simulink model "FOC_PMSM"  (Simulink 10.0)
settings: Solver=ode45  StartTime=0  StopTime=10  FixedStep=1/fs/4  MaxStep=1/fs/2  RelTol=1e-7  EnableMultiTasking=on
InitFcn:
  | Motor_parameters_Lsrpm7fw
values from neighbouring files (symbols this model uses):
  c2 = -L2/(L1^2-L2^2)    (= 10.9375)    [Motor_parameters_Lsrpm7fw.m]
  fs = 10e3    (= 10000)    [Motor_parameters_Lsrpm7fw.m]
  Iphmax = I_rated*sqrt(2)*3    [Motor_parameters_Lsrpm7fw.m]
  J = 1*1e-3    (= 0.001)    [Motor_parameters_Lsrpm7fw.m]
  Ki1 = 2    [Motor_parameters_Lsrpm7fw.m]
  Ki2 = 10000    [Motor_parameters_Lsrpm7fw.m]
  Ki_pll = 100    [Motor_parameters_Lsrpm7fw.m]
  Kp1 = 0.05    [Motor_parameters_Lsrpm7fw.m]
  Kp2 = 12    [Motor_parameters_Lsrpm7fw.m]
  Kp_pll = 10    [Motor_parameters_Lsrpm7fw.m]
  Ld = 10e-3    (= 0.01)    [Motor_parameters_Lsrpm7fw.m]
  Lndd_ini = Lndmpm    (= 0.412)    [Motor_parameters_Lsrpm7fw.m]
  Lndmpm = 0.412    [Motor_parameters_Lsrpm7fw.m]
  Lq = 12.8e-3    (= 0.0128)    [Motor_parameters_Lsrpm7fw.m]
  Npp = 8/2    (= 4)    [Motor_parameters_Lsrpm7fw.m]
  Omegae_ini = 0    [Motor_parameters_Lsrpm7fw.m]
  Rs = 0.78    [Motor_parameters_Lsrpm7fw.m]
  Tl_const = Trat/nrat^2    (= 1.24081632653e-05)    [Motor_parameters_Lsrpm7fw.m]
  Trat = 38    [Motor_parameters_Lsrpm7fw.m]
  Vm = 45    [Motor_parameters_Lsrpm7fw.m]
  Vph = Vs*sqrt(2)    [Motor_parameters_Lsrpm7fw.m]
  wo = 10    [Motor_parameters_Lsrpm7fw.m]
undefined symbols (not defined in the file or in its folder): DiscIntNeverNeededParam, sigbuilder_block
libraries: simulink x1
(part 1 of 2)
settings Model: Creator=klu  LastModifiedBy=Kristina
settings DataIOCC: LimitDataPoints=on  SignalLoggingSaveFormat=ModelDataLogs
settings OptimizationCC: BooleanDataType=off  ExpressionDepthLimit=2147483647  InitFltsAndDblsToZero=on
settings DebuggingCC: AlgebraicLoopMsg=none  SaveWithParameterizedLinksMsg=none  SignalResolutionControl=TryResolveAllWithWarning  MultiTaskDSMMsg=warning  MultiTaskCondExecSysMsg=none  FcnCallInpInsideContextMsg=warning  StateNameClashWarn=warning
settings GRTTargetCC: TargetFcnLib=ansi_tfl_tmw.mat  GeneratePreprocessorConditionals=Disable all
settings ConfigComp: CovExternalEMLEnable=off  CovSFcnEnable=off

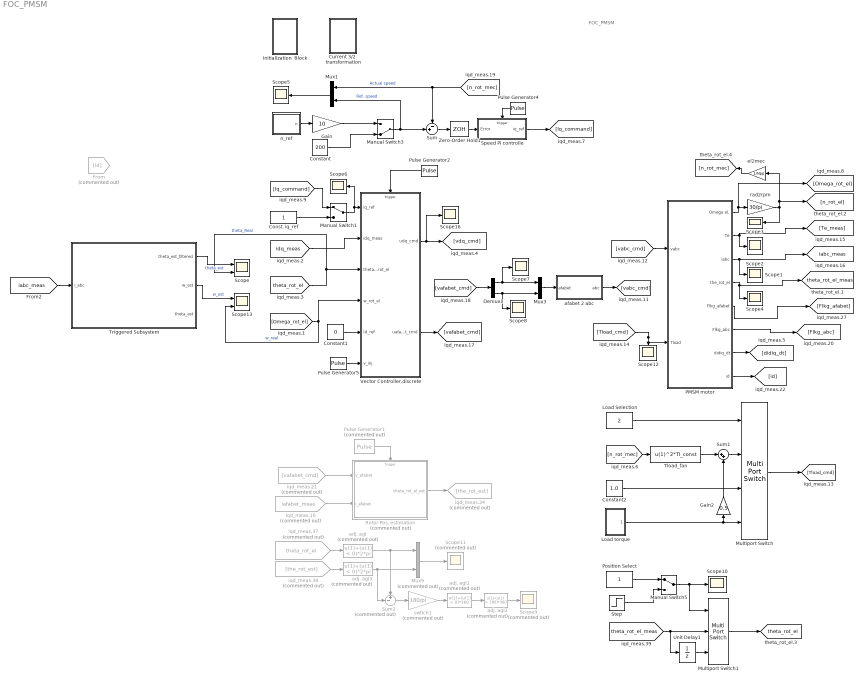
== system FOC_PMSM ==
  note: FOC_PMSM
  Const. iq_ref : Constant
  Constant : Constant  Value=200
  Constant1 : Constant  Value=0
  Constant2 : Constant  Value=1.0
  Current 3/2  transformation : Subsystem
      mask Display:
      | plot([0.1000    0.1357    0.1714    0.2071    0.2429    0.2786    0.3143    0.3500    0.3857    0.4214 0.4571    0.4929    0.5286    0.5643    0.6000]-0.05,0.4+0.6*[0.5000    0.5868    0.6564    0.6950    0.6950    0.6564    0.5868    0.5000    0.4132    0.3436 0.3050    0.3050    0.3436    0.4132    0.5000])
      | 
      | plot([0.1,0.9],[0.1,0.9])
      | 
      | plot([0.5,0.9],0.3*[1 1])
  Demux1 : Demux  Outputs=2
  From : From  Commented=on  GotoTag=id
  Gain : Gain  Gain=10
  Gain2 : Gain  Gain=0.5
  Initialization  Block : Subsystem  mask{init_in=Motor_parameters_Lsrpm7fw}
      mask prompts: init_in "Enter Initialization Script:"
      mask init:
      | aaa =3;
      mask Callback init_in:
      | init_script=get_param(gcb,'MaskValueString');
      | %eval(init_script);
      | %set_param(gcs,'PreLoadFcn',init_script)
      | set_param(gcs,'InitFcn',init_script)
      | 
      | % Change the parameters here;
      | Ld               = Ld;
      | Lq               = Ld;
  Load Selection : Constant  Value=2
  Load torque : Subsystem
  Manual Switch1 : ManualSwitch
  Manual Switch3 : ManualSwitch  CurrentSetting=0
  Manual Switch5 : ManualSwitch
  Multiport Switch : MultiPortSwitch
  Multiport Switch1 : MultiPortSwitch  Inputs=2
  Mux1 : Mux  Inputs=2
  Mux3 : Mux  Inputs=2
  Mux9 : Mux  Commented=on  Inputs=2
  PMSM motor : Subsystem
  Position Select : Constant
  Pulse Generator1 : DiscretePulseGenerator  Commented=on  PulseType=Time based  Period=1/fs  PulseWidth=50  PhaseDelay=1/fs/4*0
  Pulse Generator2 : DiscretePulseGenerator  PulseType=Time based  Period=1/fs  PulseWidth=50
  Pulse Generator4 : DiscretePulseGenerator  PulseType=Time based  Period=1/fs*2  PulseWidth=50
  Pulse Generator5 : DiscretePulseGenerator  PulseType=Time based  Amplitude=Vm  Period=2/fs  PulseWidth=50  PhaseDelay=1/fs
  Rotor Pos. estimation : Subsystem  Commented=on
  Scope : Scope  NumInputPorts=2
  Scope{1..8,10,12,16} (11 alike) : Scope
  Scope11 : Scope  Commented=on
  Scope13 : Scope  NumInputPorts=2
  Scope9 : Scope  Commented=on
  Speed PI controlle : Subsystem
  Step : Step  Time=0  Before=1  After=2  SampleTime=0
  Sum : Sum  Inputs=-+|
  Sum1 : Sum  Inputs=|++
  Sum2 : Sum  Commented=on  Inputs=+-|
  Tload_fan : Fcn  Expr=u(1)^2*Tl_const
  Triggered Subsystem : Subsystem  TreatAsAtomicUnit=on
  Unit Delay1 : UnitDelay  SampleTime=(1/fs)*4  HasFrameUpgradeWarning=on
  Vector Controller.discrete : Subsystem
  Zero-Order Hold1 : ZeroOrderHold  SampleTime=1/5e3
  adj. agl : Fcn  Commented=on  Expr=u(1)+(u(1) < 0)*2*pi
  adj. agl1 : Fcn  Commented=on  Expr=u(1)+(u(1) < 0)*360
  adj. agl2 : Fcn  Commented=on  Expr=u(1)-(u(1) > 180)*360
  adj. agl3 : Fcn  Commented=on  Expr=u(1)+(u(1) < 0)*2*pi
  afabet 2 abc : Subsystem
  el2mec : Gain  Gain=1/Npp
  iqd_meas.10 : From  Commented=on  GotoTag=iafabet_meas  TagVisibility=global
      settings: CloseFcn=tagdialog Close
  iqd_meas.21 : From  Commented=on  GotoTag=vafabet_cmd
      settings: CloseFcn=tagdialog Close
  iqd_meas.34 : Goto  Commented=on  GotoTag=the_rot_est
  iqd_meas.37 : From  Commented=on  GotoTag=theta_rot_el  TagVisibility=global
      settings: CloseFcn=tagdialog Close
  iqd_meas.38 : From  Commented=on  GotoTag=the_rot_est
      settings: CloseFcn=tagdialog Close
  n_ref : Subsystem  Tag=STV Subsys  LoadFcn=sigbuilder_block('load');  StartFcn=sigbuilder_block('start');  StopFcn=sigbuilder_block('stop');  ClipboardFcn=sigbuilder_block('clipboard');  mask(Sigbuilder block){tuvar=[0:10]}
      mask help: Sigbuilder GUI
      mask init:
      | if ~strcmp(get_param(bdroot(gcbh),'SimulationStatus'),'stopped') tuvar = sigbuilder_block('maskInit'); end
      settings: CopyFcn=sigbuilder_block('copy');  DeleteFcn=sigbuilder_block('delete');  ModelCloseFcn=sigbuilder_block('modelClose');  PreSaveFcn=sigbuilder_block('preSave');  PauseFcn=sigbuilder_block('pause')  ContinueFcn=sigbuilder_block('continue')  NameChangeFcn=sigbuilder_block('namechange');  OpenFcn=sigbuilder_block('open',[72.75 116.25 550.5 363.75 ]);  CloseFcn=sigbuilder_block('close');
      mask Display: plot(0, 0, 100, 100,[2, 2, 32, 32, 2], [68, 8, 8, 68, 68],[32, 2], [38, 38], [32, 19, 2],[53, 60, 44], [32, 17, 17, 2],[16, 16, 31, 31]);txt = getActiveGroup(gcbh);text(2, 100, txt,'verticalAlignment', 'top');
  rad2rpm : Gain  Gain=30/pi
  swtich1 : Gain  Commented=on  Gain=180/pi
  tag scope: iabc_meas=global, theta_rot_el=global, theta_rot_el_meas=global
  wires:
  Mux1/1 -> Scope5/1
  Sum/1 -> Zero-Order Hold1/1
  Manual Switch1/1 -> Scope6/1, Vector Controller.discrete/1(iq_ref)
  Const. iq_ref/1 -> Manual Switch1/2
  Zero-Order Hold1/1 -> Speed PI controlle/1(Error)
  Constant/1 -> Manual Switch3/2
  Manual Switch3/1 -> Mux1/2, Sum/2  "Ref. speed"
  [idq_meas] -> Vector Controller.discrete/2(idq_meas)
  Vector Controller.discrete/2(uafabet_cmd) -> [vafabet_cmd]
  [n_rot_mec] -> Mux1/1, Sum/1  "Actual speed"
  Constant2/1 -> Multiport Switch/3
  Load torque/1(T_load) -> Multiport Switch/4, Gain2/1
  Multiport Switch/1 -> [Tload_cmd]
  [n_rot_mec] -> Tload_fan/1
  Load Selection/1 -> Multiport Switch/1
  [theta_rot_el_meas] -> Unit Delay1/1, Multiport Switch1/2
  Multiport Switch1/1 -> [theta_rot_el]
  Position Select/1 -> Manual Switch5/1
  Step/1 -> Manual Switch5/2
  Manual Switch5/1 -> Multiport Switch1/1, Scope10/1
  n_ref/1(n) -> Gain/1
  Gain/1 -> Manual Switch3/1
  Pulse Generator2/1 -> Vector Controller.discrete/Trigger
  Sum1/1 -> Multiport Switch/2
  Tload_fan/1 -> Sum1/1
  Pulse Generator4/1 -> Speed PI controlle/Trigger
  [theta_rot_el] -> Scope/2, Vector Controller.discrete/3(theta_rot_el)  "theta_Real"
  Constant1/1 -> Vector Controller.discrete/5(Id_ref)
  Gain2/1 -> Sum1/2
  Unit Delay1/1 -> Multiport Switch1/3
  [Omega_rot_el] -> Scope13/2, Vector Controller.discrete/4(w_rot_el)  "w_real"
  PMSM motor/2(Te) -> Scope2/1, [Te_meas]
  PMSM motor/1(Omega el.) -> [Omega_rot_el], rad2rpm/1
  [vabc_cmd] -> PMSM motor/1(vabc)
  rad2rpm/1 -> el2mec/1, [n_rot_el], Scope3/1
  PMSM motor/4(the_rot_el) -> Scope4/1, [theta_rot_el_meas]
  PMSM motor/5(Flkg_afabet) -> [Flkg_afabet]
  PMSM motor/6(Flkg_abc) -> [Flkg_abc]
  [Tload_cmd] -> Scope12/1, PMSM motor/2(Tload)
  PMSM motor/3(iabc) -> Scope1/1, [iabc_meas]
  PMSM motor/7(didiq_dt) -> [didiq_dt]
  Demux1/2 -> Mux3/2, Scope8/1
  Demux1/1 -> Scope7/1, Mux3/1
  [vafabet_cmd] -> Demux1/1
  afabet 2 abc/1(abc) -> [vabc_cmd]
  Mux3/1 -> afabet 2 abc/1(afabet)
  el2mec/1 -> [n_rot_mec]
  Speed PI controlle/1(iq_ref) -> [Iq_command]
  [Iq_command] -> Manual Switch1/1
  adj. agl1/1 -> adj. agl2/1
  iqd_meas.38/1 -> adj. agl3/1
  adj. agl2/1 -> Scope9/1
  iqd_meas.10/1 -> Rotor Pos. estimation/2(i_afabet)
  swtich1/1 -> adj. agl1/1
  Sum2/1 -> swtich1/1
  iqd_meas.21/1 -> Rotor Pos. estimation/1(v_afabet)
  Mux9/1 -> Scope11/1
  Rotor Pos. estimation/1(theta_rot_el_est) -> iqd_meas.34/1
  adj. agl/1 -> Mux9/1, Sum2/1
  iqd_meas.37/1 -> adj. agl/1
  Pulse Generator1/1 -> Rotor Pos. estimation/Trigger
  adj. agl3/1 -> Mux9/2, Sum2/2
  PMSM motor/8("id   ") -> [id]
  Triggered Subsystem/2(w_est) -> Scope13/1  "w_est"
  Vector Controller.discrete/1(udq_cmd) -> Scope16/1, [vdq_cmd]
  Triggered Subsystem/1(theta_est_filtered) -> Scope/1  "theta_est"
  Pulse Generator5/1 -> Vector Controller.discrete/6("v_inj ")
  [iabc_meas] -> Triggered Subsystem/1(i_abc)

== system FOC_PMSM/Current 3/2  transformation ==
  Detect peak : Subsystem
  Display : Display
  Display1 : Display
  Manual Switch7 : ManualSwitch  CurrentSetting=0
  Scope14 : Scope
  Scope6 : Scope
  abc 2 dq : Subsystem
  dq 2 afa beta : Subsystem
  tag scope: iafabet_meas=global, idq_meas=global
  wires:
  abc 2 dq/1(dq) -> [idq_meas], Scope6/1, dq 2 afa beta/1(dq)
  dq 2 afa beta/1(afa beta) -> [iafabet_meas], Scope14/1
  Manual Switch7/1 -> abc 2 dq/1(abc), Detect peak/1(iabc)
  Detect peak/1(Peak) -> Display/1
  [theta_rot_el] -> abc 2 dq/2(theta), dq 2 afa beta/2(theta), Display1/1
  [iabc_meas] -> Manual Switch7/1, Manual Switch7/2

== system FOC_PMSM/Initialization  Block ==

== system FOC_PMSM/Load torque ==
  Add : Sum  Inputs=+++
  Scope2 : Scope
  Step Load torque 1 : Step  Time=2  After=Trat  SampleTime=0
  Step Load torque2 : Step  Time=4  After=-Trat/2  SampleTime=0
  Tload : Constant  Value=0
  T_load : Outport  VectorParamsAs1DForOutWhenUnconnected=off
  wires:
  Tload/1 -> Add/1
  Step Load torque 1/1 -> Add/2
  Step Load torque2/1 -> Add/3
  Add/1 -> T_load/1, Scope2/1

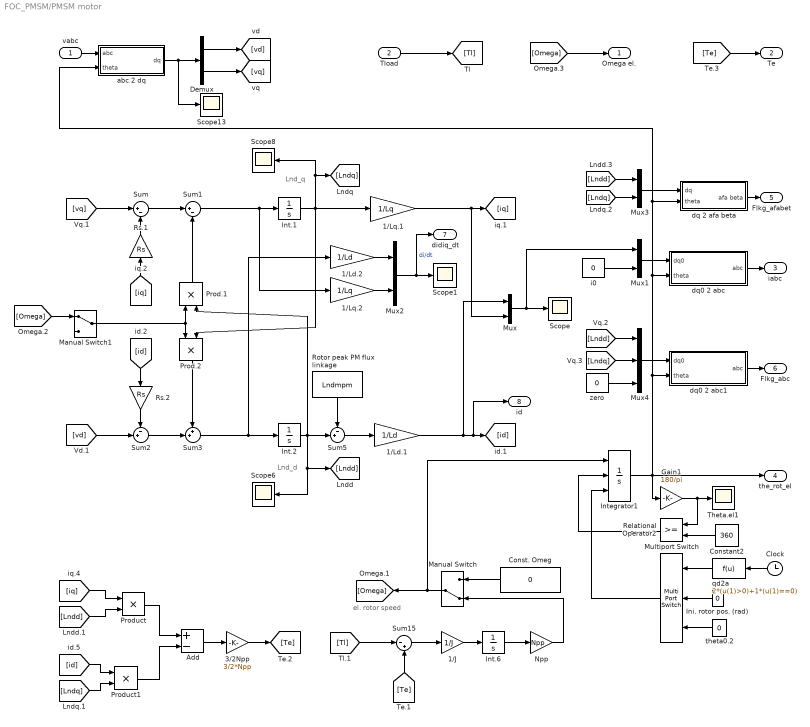
== system FOC_PMSM/PMSM motor ==
  note: Lnd_d
  note: Lnd_q
  note: el. rotor speed
  vabc : Inport
  Tload : Inport  Port=2
  1/J : Gain  Gain=1/J
  1/Ld.1 : Gain  Gain=1/Ld
  1/Ld.2 : Gain  Gain=1/Ld
  1/Lq.1 : Gain  Gain=1/Lq
  1/Lq.2 : Gain  Gain=1/Lq
  3/2Npp : Gain  Gain=3/2*Npp
  Add : Sum  Inputs=+-
  Clock : Clock
  Const. Omeg : Constant  Value=0
  Constant2 : Constant  Value=360
  Demux : Demux  Outputs=2
  Gain1 : Gain  Gain=180/pi
  Ini. rotor pos. (rad) : Constant  Value=0
  Int.1 : Integrator
  Int.2 : Integrator  InitialCondition=Lndd_ini
  Int.6 : Integrator  InitialCondition=Omegae_ini/Npp
  Integrator1 : Integrator  ExternalReset=rising  InitialConditionSource=external  InitialCondition=pi/3
  Manual Switch : ManualSwitch  CurrentSetting=0
  Manual Switch1 : ManualSwitch
  Multiport Switch : MultiPortSwitch  Inputs=2
  Mux{,1..3} (4 alike) : Mux  Inputs=2
  Mux4 : Mux  Inputs=3
  Npp : Gain  Gain=Npp
  Prod.1 : Product  RndMeth=Zero
  Prod.2 : Product  RndMeth=Zero
  Product : Product  RndMeth=Zero
  Product1 : Product  RndMeth=Zero
  Relational Operator2 : RelationalOperator  OutDataTypeStr=boolean  RndMeth=Nearest
  Rotor peak PM flux linkage : Constant  Value=Lndmpm
  Rs.1 : Gain  Gain=Rs
  Rs.2 : Gain  Gain=Rs
  Scope{,1,6,8,13} (5 alike) : Scope
  Sum : Sum  Inputs=|+-
  Sum1 : Sum  Inputs=|+-
  Sum15 : Sum  Inputs=|-+
  Sum2 : Sum  Inputs=-+|
  Sum3 : Sum  Inputs=++|
  Sum5 : Sum  Inputs=-+|
  Theta.el1 : Scope
  abc 2 dq : Subsystem
  dq 2 afa beta : Subsystem
  dq0 2 abc : Subsystem
  dq0 2 abc1 : Subsystem
  i0 : Constant  Value=0
  qd2a : Fcn  Expr=2*(u(1)>0)+1*(u(1)==0)
  theta0.2 : Constant  Value=0
  zero : Constant  Value=0
  Omega el. : Outport  VectorParamsAs1DForOutWhenUnconnected=off
  Te : Outport  Port=2  VectorParamsAs1DForOutWhenUnconnected=off
  iabc : Outport  Port=3  VectorParamsAs1DForOutWhenUnconnected=off
  the_rot_el : Outport  Port=4  VectorParamsAs1DForOutWhenUnconnected=off
  Flkg_afabet : Outport  Port=5  VectorParamsAs1DForOutWhenUnconnected=off
  Flkg_abc : Outport  Port=6  VectorParamsAs1DForOutWhenUnconnected=off
  didiq_dt : Outport  Port=7  VectorParamsAs1DForOutWhenUnconnected=off
  "id   " : Outport  Port=8  VectorParamsAs1DForOutWhenUnconnected=off
  wires:
  3/2Npp/1 -> [Te]
  Add/1 -> 3/2Npp/1
  Sum5/1 -> 1/Ld.1/1
  Rotor peak PM flux linkage/1 -> Sum5/1
  [Omega] -> Omega el./1
  [Te] -> Te/1
  Product1/1 -> Add/2
  Product/1 -> Add/1
  [Lndq] -> Product1/2
  [id] -> Product1/1
  [Te] -> Sum15/2
  Int.6/1 -> Npp/1
  1/J/1 -> Int.6/1
  Sum15/1 -> 1/J/1
  [Tl] -> Sum15/1
  Mux/1 -> Scope/1, Mux1/1
  Sum3/1 -> Int.2/1, 1/Ld.2/1
  Prod.2/1 -> Sum3/1
  Sum2/1 -> Sum3/2
  [id] -> Rs.2/1
  Rs.2/1 -> Sum2/1
  [vd] -> Sum2/2
  Int.2/1 -> [Lndd], Scope6/1, Sum5/2, Prod.1/2
  [iq] -> Rs.1/1
  Prod.1/1 -> Sum1/2
  Sum1/1 -> Int.1/1, 1/Lq.2/1
  Int.1/1 -> 1/Lq.1/1, Prod.2/2, Scope8/1, [Lndq]
  Sum/1 -> Sum1/1
  Rs.1/1 -> Sum/2
  [vq] -> Sum/1
  Tload/1 -> [Tl]
  Demux/2 -> [vq]
  Demux/1 -> [vd]
  i0/1 -> Mux1/2
  Mux1/1 -> dq0 2 abc/1(dq0)
  dq0 2 abc/1(abc) -> iabc/1
  vabc/1 -> abc 2 dq/1(abc)
  abc 2 dq/1(dq) -> Demux/1, Scope13/1
  Integrator1/1 -> the_rot_el/1, dq0 2 abc/2(theta), dq 2 afa beta/2(theta), abc 2 dq/2(theta), dq0 2 abc1/2(theta), Gain1/1
  1/Ld.2/1 -> Mux2/1
  1/Lq.2/1 -> Mux2/2
  Mux2/1 -> didiq_dt/1, Scope1/1  "di/dt"
  Mux3/1 -> dq 2 afa beta/1(dq)
  [Lndd] -> Mux3/1
  [Lndq] -> Mux3/2
  dq 2 afa beta/1(afa beta) -> Flkg_afabet/1
  [Lndd] -> Mux4/1
  [Lndq] -> Mux4/2
  Mux4/1 -> dq0 2 abc1/1(dq0)
  dq0 2 abc1/1(abc) -> Flkg_abc/1
  zero/1 -> Mux4/3
  Gain1/1 -> Theta.el1/1, Relational Operator2/1
  Constant2/1 -> Relational Operator2/2
  [iq] -> Product/1
  [Lndd] -> Product/2
  Relational Operator2/1 -> Integrator1/2
  Ini. rotor pos. (rad)/1 -> Multiport Switch/2
  theta0.2/1 -> Multiport Switch/3
  qd2a/1 -> Multiport Switch/1
  Clock/1 -> qd2a/1
  Multiport Switch/1 -> Integrator1/3
  Const. Omeg/1 -> Manual Switch/1
  Npp/1 -> Manual Switch/2
  Manual Switch/1 -> Integrator1/1, [Omega]
  [Omega] -> Manual Switch1/1
  Manual Switch1/1 -> Prod.2/1, Prod.1/1
  1/Lq.1/1 -> [iq], Mux/2
  1/Ld.1/1 -> "id   "/1, [id], Mux/1

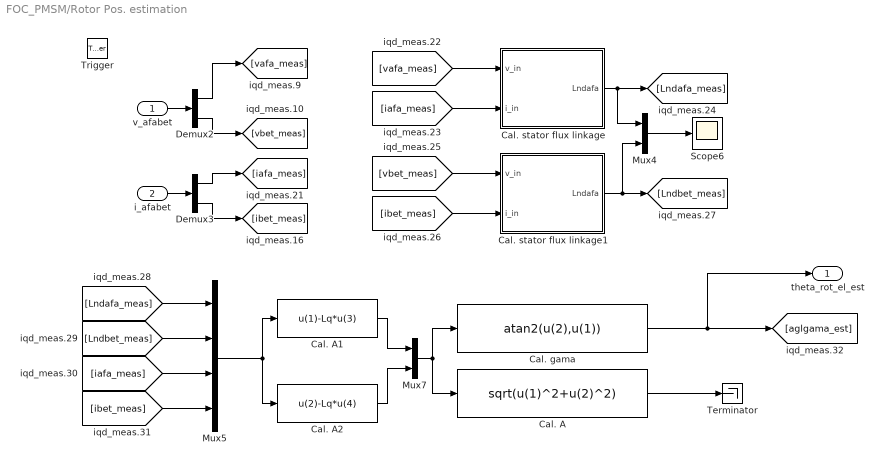
== system FOC_PMSM/Rotor Pos. estimation ==
  v_afabet : Inport  LatchByDelayingOutsideSignal=on
  i_afabet : Inport  Port=2  LatchByDelayingOutsideSignal=on
  Trigger : TriggerPort  VariantControl=(inherit)
  Cal. A : Fcn  Expr=sqrt(u(1)^2+u(2)^2)
  Cal. A1 : Fcn  Expr=u(1)-Lq*u(3)
  Cal. A2 : Fcn  Expr=u(2)-Lq*u(4)
  Cal. gama : Fcn  Expr=atan2(u(2),u(1))
  Cal. stator flux linkage : Subsystem
  Cal. stator flux linkage1 : Subsystem
  Demux2 : Demux  Outputs=2
  Demux3 : Demux  Outputs=2
  Mux4 : Mux  Inputs=2
  Mux5 : Mux
  Mux7 : Mux  Inputs=2
  Scope6 : Scope
  Terminator : Terminator
  theta_rot_el_est : Outport  VectorParamsAs1DForOutWhenUnconnected=off
  wires:
  Demux2/1 -> [vafa_meas]
  Demux2/2 -> [vbet_meas]
  Demux3/1 -> [iafa_meas]
  Demux3/2 -> [ibet_meas]
  [vafa_meas] -> Cal. stator flux linkage/1(v_in)
  [iafa_meas] -> Cal. stator flux linkage/2(i_in)
  Cal. stator flux linkage/1(Lndafa) -> [Lndafa_meas], Mux4/1
  [vbet_meas] -> Cal. stator flux linkage1/1(v_in)
  [ibet_meas] -> Cal. stator flux linkage1/2(i_in)
  Cal. stator flux linkage1/1(Lndafa) -> [Lndbet_meas], Mux4/2
  Mux4/1 -> Scope6/1
  [Lndafa_meas] -> Mux5/1
  [Lndbet_meas] -> Mux5/2
  [iafa_meas] -> Mux5/3
  [ibet_meas] -> Mux5/4
  Mux5/1 -> Cal. A1/1, Cal. A2/1
  Cal. A1/1 -> Mux7/1
  Cal. A2/1 -> Mux7/2
  Mux7/1 -> Cal. gama/1, Cal. A/1
  Cal. A/1 -> Terminator/1
  v_afabet/1 -> Demux2/1
  i_afabet/1 -> Demux3/1
  Cal. gama/1 -> theta_rot_el_est/1, [aglgama_est]

== system FOC_PMSM/Speed PI controlle ==
  Error : Inport
  Trigger : TriggerPort  VariantControl=(inherit)
  Discrete-Time Integrator : DiscreteIntegrator  SampleTime=-1  ICPrevOutput=DiscIntNeverNeededParam  ICPrevScaledInput=DiscIntNeverNeededParam
  Kp : Gain  Gain=Kp1
  Sum1 : Sum  Inputs=|++
  ki : Gain  Gain=Ki1
  iq_ref : Outport  VectorParamsAs1DForOutWhenUnconnected=off
  wires:
  Kp/1 -> Sum1/1
  ki/1 -> Discrete-Time Integrator/1
  Discrete-Time Integrator/1 -> Sum1/2
  Sum1/1 -> iq_ref/1
  Error/1 -> Kp/1, ki/1

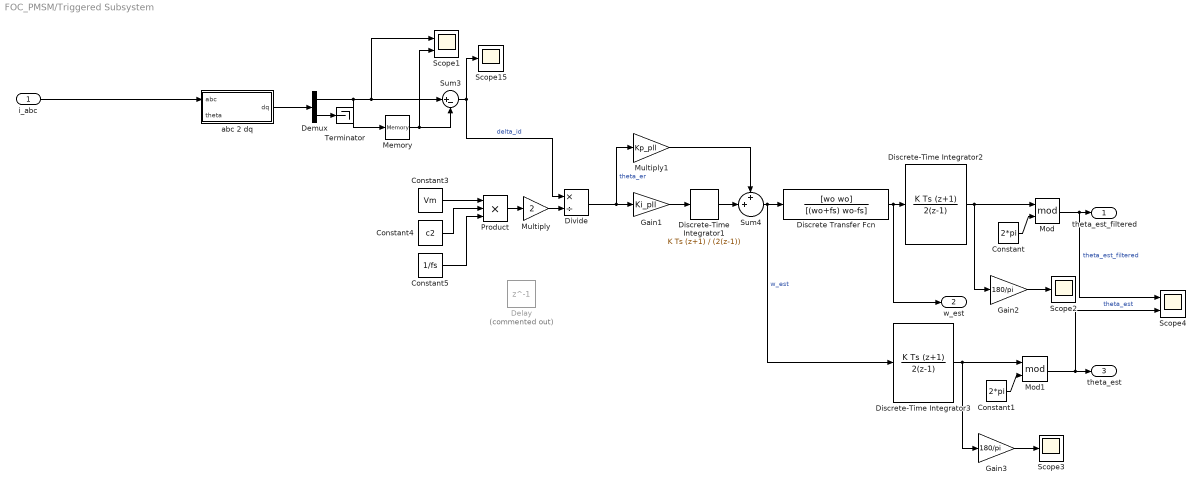
== system FOC_PMSM/Triggered Subsystem ==
  i_abc : Inport
  Constant : Constant  Value=2*pi
  Constant1 : Constant  Value=2*pi
  Constant3 : Constant  Value=Vm
  Constant4 : Constant  Value=c2
  Constant5 : Constant  Value=1/fs
  Delay : Delay  Commented=on  DelayLength=1
  Demux : Demux  Outputs=2
  Discrete Transfer Fcn : DiscreteTransferFcn  Numerator=[wo wo]  Denominator=[(wo+fs) wo-fs]
  Discrete-Time Integrator1 : DiscreteIntegrator  IntegratorMethod=Integration: Trapezoidal  gainval=1  InitialCondition=83  SampleTime=-1  ICPrevOutput=DiscIntNeverNeededParam  ICPrevScaledInput=DiscIntNeverNeededParam
  Discrete-Time Integrator2 : DiscreteIntegrator  IntegratorMethod=Integration: Trapezoidal  gainval=1  SampleTime=-1  ICPrevOutput=DiscIntNeverNeededParam  ICPrevScaledInput=DiscIntNeverNeededParam
  Discrete-Time Integrator3 : DiscreteIntegrator  IntegratorMethod=Integration: Trapezoidal  gainval=1  SampleTime=-1  ICPrevOutput=DiscIntNeverNeededParam  ICPrevScaledInput=DiscIntNeverNeededParam
  Divide : Product  Inputs=*/
  Gain1 : Gain  Gain=Ki_pll
  Gain2 : Gain  Gain=180/pi
  Gain3 : Gain  Gain=180/pi
  Memory : Memory  InheritSampleTime=on
  Mod : Math  Operator=mod  SignedPower=off  SaturateOnIntegerOverflow=on
  Mod1 : Math  Operator=mod  SignedPower=off  SaturateOnIntegerOverflow=on
  Multiply : Gain  Gain=2
  Multiply1 : Gain  Gain=Kp_pll
  Product : Product  Inputs=3
  Scope1 : Scope  NumInputPorts=2
  Scope15 : Scope
  Scope2 : Scope
  Scope3 : Scope
  Scope4 : Scope  NumInputPorts=2
  Sum3 : Sum  Inputs=|+-
  Sum4 : Sum  Inputs=++|
  Terminator : Terminator
  abc 2 dq : Subsystem
  theta_est_filtered : Outport
  w_est : Outport  Port=2
  theta_est : Outport  Port=3
  wires:
  Constant3/1 -> Product/1
  Constant4/1 -> Product/2
  Gain1/1 -> Discrete-Time Integrator1/1
  Divide/1 -> Multiply1/1, Gain1/1  "theta_er"
  Discrete-Time Integrator1/1 -> Sum4/2
  Multiply1/1 -> Sum4/1
  Multiply/1 -> Divide/2
  Constant5/1 -> Product/3
  Product/1 -> Multiply/1
  Gain2/1 -> Scope2/1
  Discrete-Time Integrator2/1 -> Mod/1, Gain2/1
  Mod/1 -> Scope4/1, theta_est_filtered/1  "theta_est_filtered"
  Constant/1 -> Mod/2
  Memory/1 -> Sum3/2, Scope1/2
  Demux/1 -> Sum3/1, Scope1/1, Memory/1
  Sum3/1 -> Scope15/1, Divide/1  "delta_id"
  i_abc/1 -> abc 2 dq/1(abc)
  abc 2 dq/1(dq) -> Demux/1
  Demux/2 -> Terminator/1
  Sum4/1 -> Discrete-Time Integrator3/1, Discrete Transfer Fcn/1  "w_est"
  Discrete Transfer Fcn/1 -> w_est/1, Discrete-Time Integrator2/1
  Discrete-Time Integrator3/1 -> Mod1/1, Gain3/1
  Mod1/1 -> Scope4/2, theta_est/1  "theta_est"
  Gain3/1 -> Scope3/1
  Constant1/1 -> Mod1/2

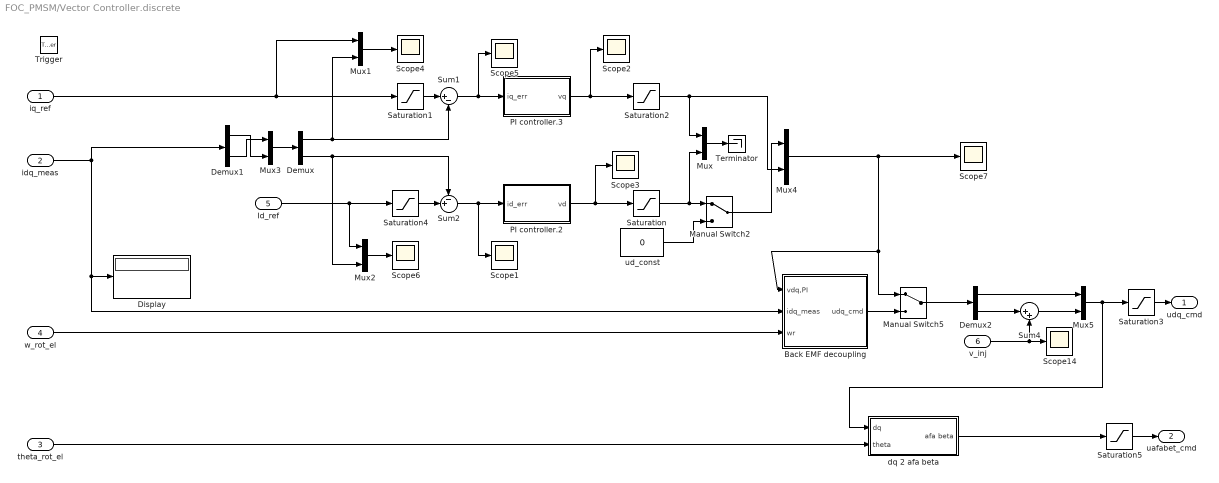
== system FOC_PMSM/Vector Controller.discrete ==
  iq_ref : Inport
  idq_meas : Inport  Port=2
  theta_rot_el : Inport  Port=3
  w_rot_el : Inport  Port=4
  Id_ref : Inport  Port=5
  "v_inj " : Inport  Port=6
  Trigger : TriggerPort  VariantControl=(inherit)
  Back EMF decoupling : Subsystem
  Demux : Demux  Outputs=2
  Demux1 : Demux  Outputs=2
  Demux2 : Demux  Outputs=2
  Display : Display
  Manual Switch2 : ManualSwitch
  Manual Switch5 : ManualSwitch
  Mux{,1..5} (6 alike) : Mux  Inputs=2
  PI controller.2 : Subsystem
  PI controller.3 : Subsystem
  Saturation{,2..3,5} (4 alike) : Saturate  UpperLimit=Vph  LowerLimit=-Vph
  Saturation1 : Saturate  UpperLimit=Iphmax  LowerLimit=-Iphmax
  Saturation4 : Saturate  UpperLimit=Iphmax  LowerLimit=-Iphmax
  Scope{1..7,14} (8 alike) : Scope
  Sum1 : Sum  Inputs=|+-
  Sum2 : Sum  Inputs=-+|
  Sum4 : Sum  Inputs=|++
  Terminator : Terminator
  dq 2 afa beta : Subsystem
  ud_const : Constant  Value=0
  udq_cmd : Outport  VectorParamsAs1DForOutWhenUnconnected=off
  uafabet_cmd : Outport  Port=2  VectorParamsAs1DForOutWhenUnconnected=off
  wires:
  Saturation4/1 -> Sum2/2
  Saturation/1 -> Mux/2, Manual Switch2/1
  Mux/1 -> Terminator/1
  PI controller.3/1(vq) -> Scope2/1, Saturation2/1
  Demux/1 -> Sum1/2, Mux1/2
  PI controller.2/1(vd) -> Saturation/1, Scope3/1
  Demux/2 -> Sum2/1, Mux2/2
  Sum1/1 -> Scope5/1, PI controller.3/1(iq_err)
  iq_ref/1 -> Mux1/1, Saturation1/1
  Sum2/1 -> Scope1/1, PI controller.2/1(id_err)
  Id_ref/1 -> Saturation4/1, Mux2/1
  Mux1/1 -> Scope4/1
  Saturation1/1 -> Sum1/1
  Mux2/1 -> Scope6/1
  Saturation2/1 -> Mux/1, Mux4/2
  Manual Switch2/1 -> Mux4/1
  ud_const/1 -> Manual Switch2/2
  Demux1/2 -> Mux3/1
  Demux1/1 -> Mux3/2
  theta_rot_el/1 -> dq 2 afa beta/2(theta)
  dq 2 afa beta/1(afa beta) -> Saturation5/1
  w_rot_el/1 -> Back EMF decoupling/3(wr)
  Back EMF decoupling/1(udq_cmd) -> Manual Switch5/2
  Mux4/1 -> Scope7/1, Manual Switch5/1, Back EMF decoupling/1(vdq,PI)
  Mux3/1 -> Demux/1
  idq_meas/1 -> Demux1/1, Display/1, Back EMF decoupling/2(idq_meas)
  Saturation3/1 -> udq_cmd/1
  Saturation5/1 -> uafabet_cmd/1
  Manual Switch5/1 -> Demux2/1
  Sum4/1 -> Mux5/2
  "v_inj "/1 -> Scope14/1, Sum4/2
  Mux5/1 -> dq 2 afa beta/1(dq), Saturation3/1
  Demux2/2 -> Sum4/1
  Demux2/1 -> Mux5/1

== system FOC_PMSM/afabet 2 abc ==
  afabet : Inport
  Constant : Constant  Value=0
  Mux1 : Mux  Inputs=2
  Mux2 : Mux  Inputs=3
  qd2a : Fcn  Expr=u(1)+u(3)
  qd2b : Fcn  Expr=u(1)*cos(2/3*pi)+u(2)*sin(2/3*pi)+u(3)
  qd2c : Fcn  Expr=u(1)*cos(2/3*pi)-u(2)*sin(2/3*pi)+u(3)
  abc : Outport  VectorParamsAs1DForOutWhenUnconnected=off
  wires:
  Constant/1 -> Mux1/2
  qd2c/1 -> Mux2/3
  afabet/1 -> Mux1/1
  Mux1/1 -> qd2c/1, qd2b/1, qd2a/1
  qd2a/1 -> Mux2/1
  qd2b/1 -> Mux2/2
  Mux2/1 -> abc/1

== system FOC_PMSM/n_ref ==
  Demux : Demux  Tag=STV Demux  Outputs=1
  FromWs : FromWorkspace  Tag=STV FromWs  VariableName=tuvar  SampleTime=0  SigBuilderData=DataTag0  VnvData=DataTag1
      SigBuilderData=|
      | common.afterFinalStr = 'Extrapolate'
      | common.sampleTime = 0
      | dataSet.timeRange = [0 10]
      | dataSet.name = 'Group 1'
      | sbobj.Groups.Name = 'Group 1'
      | sbobj.Groups.Signals.Name = 'n'
      | sbobj.Groups.Signals.XData = [0 1 1 6 7 10]
      | sbobj.Groups.Signals.YData = [0 0 1 1 0.39 0.1]
  n : Outport  Tag=STV Outport  VectorParamsAs1DForOutWhenUnconnected=off
  wires:
  Demux/1 -> n/1
  FromWs/1 -> Demux/1

== system FOC_PMSM/Current 3/2  transformation/Detect peak ==
  iabc : Inport
  Clock : Clock
  Compare To Constant : simulink/Logic and Bit Operations/Compare To Constant  relop=>=  const=2  OutDataTypeStr=uint8  ZeroCross=off
  Demux1 : Demux  Outputs=3
  MinMax : MinMax  Function=max  Inputs=2
  Product : Product  RndMeth=Zero
  Terminator : Terminator
  Terminator1 : Terminator
  Unit Delay : UnitDelay  SampleTime=1/5e3  HasFrameUpgradeWarning=on
  Peak : Outport  VectorParamsAs1DForOutWhenUnconnected=off
  wires:
  iabc/1 -> Demux1/1
  Demux1/3 -> Terminator/1
  Demux1/2 -> Terminator1/1
  Clock/1 -> Compare To Constant/1
  Compare To Constant/1 -> Product/1
  Demux1/1 -> Product/2
  MinMax/1 -> Peak/1, Unit Delay/1
  Product/1 -> MinMax/1
  Unit Delay/1 -> MinMax/2

== system FOC_PMSM/Current 3/2  transformation/abc 2 dq ==
  abc : Inport
  theta : Inport  Port=2
  Mux1 : Mux  Inputs=2
  Mux2 : Mux  Inputs=2
  abc2d : Fcn  Expr=2/3*(u(1)*cos(u(4))+u(2)*cos(u(4)-2*pi/3)+u(3)*cos(u(4)-4*pi/3))
  abc2q : Fcn  Expr=-1*2/3*(u(1)*sin(u(4))+u(2)*sin(u(4)-2*pi/3)+u(3)*sin(u(4)-4*pi/3))
  dq : Outport  VectorParamsAs1DForOutWhenUnconnected=off
  wires:
  Mux2/1 -> dq/1
  abc2q/1 -> Mux2/2
  abc2d/1 -> Mux2/1
  Mux1/1 -> abc2q/1, abc2d/1
  theta/1 -> Mux1/2
  abc/1 -> Mux1/1

== system FOC_PMSM/Current 3/2  transformation/dq 2 afa beta ==
  dq : Inport
  theta : Inport  Port=2
  Mux1 : Mux  Inputs=2
  Mux2 : Mux  Inputs=2
  dq2afa : Fcn  Expr=u(1)*cos(u(3))-u(2)*sin(u(3))
  dq2beta : Fcn  Expr=u(1)*sin(u(3))+u(2)*cos(u(3))
  afa beta : Outport  VectorParamsAs1DForOutWhenUnconnected=off
  wires:
  dq/1 -> Mux1/1
  theta/1 -> Mux1/2
  Mux1/1 -> dq2beta/1, dq2afa/1
  dq2afa/1 -> Mux2/1
  dq2beta/1 -> Mux2/2
  Mux2/1 -> afa beta/1

== system FOC_PMSM/PMSM motor/abc 2 dq ==
  abc : Inport
  theta : Inport  Port=2
  Mux1 : Mux  Inputs=2
  Mux2 : Mux  Inputs=2
  abc2d : Fcn  Expr=-1*2/3*(u(1)*sin(u(4))+u(2)*sin(u(4)-2*pi/3)+u(3)*sin(u(4)-4*pi/3))
  abc2q : Fcn  Expr=2/3*(u(1)*cos(u(4))+u(2)*cos(u(4)-2*pi/3)+u(3)*cos(u(4)-4*pi/3))
  dq : Outport  VectorParamsAs1DForOutWhenUnconnected=off
  wires:
  Mux2/1 -> dq/1
  abc2d/1 -> Mux2/2
  abc2q/1 -> Mux2/1
  Mux1/1 -> abc2d/1, abc2q/1
  theta/1 -> Mux1/2
  abc/1 -> Mux1/1

== system FOC_PMSM/PMSM motor/dq 2 afa beta ==
  dq : Inport
  theta : Inport  Port=2
  Mux1 : Mux  Inputs=2
  Mux2 : Mux  Inputs=2
  dq2afa : Fcn  Expr=u(1)*cos(u(3))-u(2)*sin(u(3))
  dq2beta : Fcn  Expr=u(1)*sin(u(3))+u(2)*cos(u(3))
  afa beta : Outport  VectorParamsAs1DForOutWhenUnconnected=off
  wires:
  dq/1 -> Mux1/1
  theta/1 -> Mux1/2
  Mux1/1 -> dq2beta/1, dq2afa/1
  dq2afa/1 -> Mux2/1
  dq2beta/1 -> Mux2/2
  Mux2/1 -> afa beta/1

== system FOC_PMSM/PMSM motor/dq0 2 abc ==
  dq0 : Inport
  theta : Inport  Port=2
  Mux1 : Mux  Inputs=2
  Mux2 : Mux  Inputs=3
  qd2a : Fcn  Expr=u(1)*cos(u(4))-u(2)*sin(u(4))+u(3)
  qd2b : Fcn  Expr=u(1)*cos(u(4)-2/3*pi)-u(2)*sin(u(4)-2/3*pi)+u(3)
  qd2c : Fcn  Expr=u(1)*cos(u(4)+2/3*pi)-u(2)*sin(u(4)+2/3*pi)+u(3)
  abc : Outport  VectorParamsAs1DForOutWhenUnconnected=off
  wires:
  Mux2/1 -> abc/1
  qd2b/1 -> Mux2/2
  qd2a/1 -> Mux2/1
  Mux1/1 -> qd2b/1, qd2c/1, qd2a/1
  theta/1 -> Mux1/2
  dq0/1 -> Mux1/1
  qd2c/1 -> Mux2/3

== system FOC_PMSM/PMSM motor/dq0 2 abc1 ==
  dq0 : Inport
  theta : Inport  Port=2
  Mux1 : Mux  Inputs=2
  Mux2 : Mux  Inputs=3
  qd2a : Fcn  Expr=u(1)*cos(u(4))-u(2)*sin(u(4))+u(3)
  qd2b : Fcn  Expr=u(1)*cos(u(4)-2/3*pi)-u(2)*sin(u(4)-2/3*pi)+u(3)
  qd2c : Fcn  Expr=u(1)*cos(u(4)+2/3*pi)-u(2)*sin(u(4)+2/3*pi)+u(3)
  abc : Outport  VectorParamsAs1DForOutWhenUnconnected=off
  wires:
  qd2c/1 -> Mux2/3
  dq0/1 -> Mux1/1
  theta/1 -> Mux1/2
  Mux1/1 -> qd2a/1, qd2c/1, qd2b/1
  qd2a/1 -> Mux2/1
  qd2b/1 -> Mux2/2
  Mux2/1 -> abc/1

== system FOC_PMSM/Rotor Pos. estimation/Cal. stator flux linkage ==
  v_in : Inport
  i_in : Inport  Port=2
  Discrete-Time Integrator : DiscreteIntegrator  SampleTime=-1  ICPrevOutput=DiscIntNeverNeededParam  ICPrevScaledInput=DiscIntNeverNeededParam
  Gain : Gain  Gain=Rs/2
  MinMax detection : Subsystem
  Scope6 : Scope
  Sum1 : Sum  Inputs=|+-
  Sum2 : Sum  Inputs=|+-
  Terminator : Terminator
  Terminator1 : Terminator
  Lndafa : Outport  VectorParamsAs1DForOutWhenUnconnected=off
  wires:
  MinMax detection/3(average) -> Sum2/2, Scope6/1
  Sum2/1 -> Lndafa/1
  MinMax detection/1(max.ou) -> Terminator/1
  MinMax detection/2(min.ou) -> Terminator1/1
  Gain/1 -> Sum1/2
  v_in/1 -> Sum1/1
  i_in/1 -> Gain/1
  Sum1/1 -> Discrete-Time Integrator/1
  Discrete-Time Integrator/1 -> Sum2/1, MinMax detection/1(In)

== system FOC_PMSM/Rotor Pos. estimation/Cal. stator flux linkage1 ==
  v_in : Inport
  i_in : Inport  Port=2
  Discrete-Time Integrator : DiscreteIntegrator  SampleTime=-1  ICPrevOutput=DiscIntNeverNeededParam  ICPrevScaledInput=DiscIntNeverNeededParam
  Gain : Gain  Gain=Rs/2
  MinMax detection : Subsystem
  Scope6 : Scope
  Sum1 : Sum  Inputs=|+-
  Sum2 : Sum  Inputs=|+-
  Terminator : Terminator
  Terminator1 : Terminator
  Lndafa : Outport  VectorParamsAs1DForOutWhenUnconnected=off
  wires:
  Discrete-Time Integrator/1 -> Sum2/1, MinMax detection/1(In)
  Sum1/1 -> Discrete-Time Integrator/1
  i_in/1 -> Gain/1
  v_in/1 -> Sum1/1
  Gain/1 -> Sum1/2
  MinMax detection/2(min.ou) -> Terminator1/1
  MinMax detection/1(max.ou) -> Terminator/1
  Sum2/1 -> Lndafa/1
  MinMax detection/3(average) -> Sum2/2, Scope6/1

== system FOC_PMSM/Triggered Subsystem/abc 2 dq ==
  abc : Inport
  theta : Inport  Port=2
  Mux1 : Mux  Inputs=2
  Mux2 : Mux  Inputs=2
  abc2d : Fcn  Expr=2/3*(u(1)*cos(u(4))+u(2)*cos(u(4)-2*pi/3)+u(3)*cos(u(4)-4*pi/3))
  abc2q : Fcn  Expr=-1*2/3*(u(1)*sin(u(4))+u(2)*sin(u(4)-2*pi/3)+u(3)*sin(u(4)-4*pi/3))
  dq : Outport  VectorParamsAs1DForOutWhenUnconnected=off
  wires:
  Mux2/1 -> dq/1
  abc2q/1 -> Mux2/2
  abc2d/1 -> Mux2/1
  Mux1/1 -> abc2q/1, abc2d/1
  theta/1 -> Mux1/2
  abc/1 -> Mux1/1

== system FOC_PMSM/Vector Controller.discrete/Back EMF decoupling ==
  vdq,PI : Inport
  idq_meas : Inport  Port=2
  wr : Inport  Port=3
  Demux1 : Demux  Outputs=2
  Demux2 : Demux  Outputs=2
  Gain : Gain  Gain=Lq
  Gain1 : Gain  Gain=Ld
  Lndmpm : Constant  Value=Lndmpm
  Mux2 : Mux  Inputs=2
  Product : Product  RndMeth=Zero
  Product1 : Product  RndMeth=Zero
  Product2 : Product  RndMeth=Zero
  Sum : Sum  Inputs=|+-
  Sum1 : Sum  Inputs=|++
  Sum2 : Sum  Inputs=|++
  udq_cmd : Outport  VectorParamsAs1DForOutWhenUnconnected=off
  wires:
  Mux2/1 -> udq_cmd/1
  vdq,PI/1 -> Demux1/1
  Demux1/1 -> Sum/1
  Sum/1 -> Mux2/1
  Demux1/2 -> Sum1/1
  idq_meas/1 -> Demux2/1
  wr/1 -> Product/2, Product1/1, Product2/2
  Product1/1 -> Sum/2
  Gain/1 -> Product1/2
  Demux2/2 -> Gain/1
  Lndmpm/1 -> Product/1
  Product/1 -> Sum1/2
  Sum1/1 -> Sum2/1
  Demux2/1 -> Gain1/1
  Gain1/1 -> Product2/1
  Product2/1 -> Sum2/2
  Sum2/1 -> Mux2/2

== system FOC_PMSM/Vector Controller.discrete/PI controller.2 ==
  id_err : Inport
  Discrete-Time Integrator : DiscreteIntegrator  SampleTime=-1  ICPrevOutput=DiscIntNeverNeededParam  ICPrevScaledInput=DiscIntNeverNeededParam
  Kp : Gain  Gain=Kp2
  Sum1 : Sum  Inputs=|++
  ki : Gain  Gain=Ki2
  vd : Outport  VectorParamsAs1DForOutWhenUnconnected=off
  wires:
  Sum1/1 -> vd/1
  Discrete-Time Integrator/1 -> Sum1/2
  ki/1 -> Discrete-Time Integrator/1
  Kp/1 -> Sum1/1
  id_err/1 -> ki/1, Kp/1

== system FOC_PMSM/Vector Controller.discrete/PI controller.3 ==
  iq_err : Inport
  Discrete-Time Integrator : DiscreteIntegrator  SampleTime=-1  ICPrevOutput=DiscIntNeverNeededParam  ICPrevScaledInput=DiscIntNeverNeededParam
  Kp : Gain  Gain=8
  Sum1 : Sum  Inputs=|++
  ki : Gain  Gain=5000
  vq : Outport  VectorParamsAs1DForOutWhenUnconnected=off
  wires:
  Sum1/1 -> vq/1
  Discrete-Time Integrator/1 -> Sum1/2
  ki/1 -> Discrete-Time Integrator/1
  Kp/1 -> Sum1/1
  iq_err/1 -> ki/1, Kp/1

== system FOC_PMSM/Vector Controller.discrete/dq 2 afa beta ==
  dq : Inport
  theta : Inport  Port=2
  Mux1 : Mux  Inputs=2
  Mux2 : Mux  Inputs=2
  dq2afa : Fcn  Expr=u(1)*cos(u(3))-u(2)*sin(u(3))
  dq2beta : Fcn  Expr=u(1)*sin(u(3))+u(2)*cos(u(3))
  afa beta : Outport  VectorParamsAs1DForOutWhenUnconnected=off
  wires:
  Mux2/1 -> afa beta/1
  dq2beta/1 -> Mux2/2
  dq2afa/1 -> Mux2/1
  Mux1/1 -> dq2afa/1, dq2beta/1
  theta/1 -> Mux1/2
  dq/1 -> Mux1/1

== system FOC_PMSM/Rotor Pos. estimation/Cal. stator flux linkage/MinMax detection ==
  In : Inport
  Gain : Gain  Gain=1/2
  Max. Det : Subsystem
  Min. Det : Subsystem
  Mux6 : Mux  Inputs=3
  Scope5 : Scope
  Sum : Sum  Inputs=|++
  max.ou : Outport  VectorParamsAs1DForOutWhenUnconnected=off
  min.ou : Outport  Port=2  VectorParamsAs1DForOutWhenUnconnected=off
  average : Outport  Port=3  VectorParamsAs1DForOutWhenUnconnected=off
  wires:
  Gain/1 -> average/1
  Sum/1 -> Gain/1
  Max. Det/1(Max) -> max.ou/1, Mux6/1, Sum/1
  Min. Det/1(Min) -> min.ou/1, Mux6/3, Sum/2
  Mux6/1 -> Scope5/1
  In/1 -> Max. Det/1(In), Min. Det/1(In), Mux6/2

== system FOC_PMSM/Rotor Pos. estimation/Cal. stator flux linkage1/MinMax detection ==
  In : Inport
  Gain : Gain  Gain=1/2
  Max. Det : Subsystem
  Min. Det : Subsystem
  Mux6 : Mux  Inputs=3
  Scope5 : Scope
  Sum : Sum  Inputs=|++
  max.ou : Outport  VectorParamsAs1DForOutWhenUnconnected=off
  min.ou : Outport  Port=2  VectorParamsAs1DForOutWhenUnconnected=off
  average : Outport  Port=3  VectorParamsAs1DForOutWhenUnconnected=off
  wires:
  Gain/1 -> average/1
  Sum/1 -> Gain/1
  Max. Det/1(Max) -> max.ou/1, Mux6/1, Sum/1
  Min. Det/1(Min) -> min.ou/1, Mux6/3, Sum/2
  Mux6/1 -> Scope5/1
  In/1 -> Max. Det/1(In), Min. Det/1(In), Mux6/2

== system FOC_PMSM/Rotor Pos. estimation/Cal. stator flux linkage/MinMax detection/Max. Det ==
  In : Inport
  Counter.1 : Subsystem
  Counter.2 : Subsystem
  Gain1 : Gain
  Gain2 : Gain  Gain=0.3
  Gain3 : Gain  Gain=0.6
  Mux2 : Mux
  Product : Product  RndMeth=Zero
  Relational Operator : RelationalOperator  RndMeth=Nearest
  Scope3 : Scope
  Unit Delay : UnitDelay  SampleTime=-1  HasFrameUpgradeWarning=on
  max.1 : Subsystem
  max.3 : Subsystem
  Max : Outport  VectorParamsAs1DForOutWhenUnconnected=off
  wires:
  Unit Delay/1 -> Relational Operator/2
  In/1 -> Unit Delay/1, max.1/1(In), Relational Operator/1, Mux2/1
  Relational Operator/1 -> max.1/Trigger, Counter.1/1(Sig.In), Counter.2/1(Sig.In), Gain1/1
  max.1/1(Out) -> max.3/1(In)
  Counter.1/1(En) -> Product/2, Gain3/1
  Mux2/1 -> Scope3/1
  Counter.2/1(En) -> Product/1, Gain2/1
  Product/1 -> max.3/Trigger
  Gain1/1 -> Mux2/2
  Gain2/1 -> Mux2/3
  Gain3/1 -> Mux2/4
  max.3/1(Out) -> Max/1

== system FOC_PMSM/Rotor Pos. estimation/Cal. stator flux linkage/MinMax detection/Min. Det ==
  In : Inport
  Counter.1 : Subsystem
  Counter.2 : Subsystem
  Gain1 : Gain
  Gain2 : Gain  Gain=0.3
  Gain3 : Gain  Gain=0.6
  Mux2 : Mux
  Product : Product  RndMeth=Zero
  Relational Operator : RelationalOperator  Operator=<=  RndMeth=Nearest
  Scope3 : Scope
  Unit Delay : UnitDelay  SampleTime=-1  HasFrameUpgradeWarning=on
  max.1 : Subsystem
  max.3 : Subsystem
  Min : Outport  VectorParamsAs1DForOutWhenUnconnected=off
  wires:
  max.3/1(Out) -> Min/1
  Gain3/1 -> Mux2/4
  Gain2/1 -> Mux2/3
  Gain1/1 -> Mux2/2
  Product/1 -> max.3/Trigger
  Counter.2/1(En) -> Gain2/1, Product/1
  Mux2/1 -> Scope3/1
  Counter.1/1(En) -> Gain3/1, Product/2
  max.1/1(Out) -> max.3/1(In)
  Relational Operator/1 -> Gain1/1, Counter.2/1(Sig.In), Counter.1/1(Sig.In), max.1/Trigger
  In/1 -> Mux2/1, Relational Operator/1, max.1/1(In), Unit Delay/1
  Unit Delay/1 -> Relational Operator/2

== system FOC_PMSM/Rotor Pos. estimation/Cal. stator flux linkage1/MinMax detection/Max. Det ==
  In : Inport
  Counter.1 : Subsystem
  Counter.2 : Subsystem
  Gain1 : Gain
  Gain2 : Gain  Gain=0.3
  Gain3 : Gain  Gain=0.6
  Mux2 : Mux
  Product : Product  RndMeth=Zero
  Relational Operator : RelationalOperator  RndMeth=Nearest
  Scope3 : Scope
  Unit Delay : UnitDelay  SampleTime=-1  HasFrameUpgradeWarning=on
  max.1 : Subsystem
  max.3 : Subsystem
  Max : Outport  VectorParamsAs1DForOutWhenUnconnected=off
  wires:
  Unit Delay/1 -> Relational Operator/2
  In/1 -> Unit Delay/1, max.1/1(In), Relational Operator/1, Mux2/1
  Relational Operator/1 -> max.1/Trigger, Counter.1/1(Sig.In), Counter.2/1(Sig.In), Gain1/1
  max.1/1(Out) -> max.3/1(In)
  Counter.1/1(En) -> Product/2, Gain3/1
  Mux2/1 -> Scope3/1
  Counter.2/1(En) -> Product/1, Gain2/1
  Product/1 -> max.3/Trigger
  Gain1/1 -> Mux2/2
  Gain2/1 -> Mux2/3
  Gain3/1 -> Mux2/4
  max.3/1(Out) -> Max/1

== system FOC_PMSM/Rotor Pos. estimation/Cal. stator flux linkage1/MinMax detection/Min. Det ==
  In : Inport
  Counter.1 : Subsystem
  Counter.2 : Subsystem
  Gain1 : Gain
  Gain2 : Gain  Gain=0.3
  Gain3 : Gain  Gain=0.6
  Mux2 : Mux
  Product : Product  RndMeth=Zero
  Relational Operator : RelationalOperator  Operator=<=  RndMeth=Nearest
  Scope3 : Scope
  Unit Delay : UnitDelay  SampleTime=-1  HasFrameUpgradeWarning=on
  max.1 : Subsystem
  max.3 : Subsystem
  Min : Outport  VectorParamsAs1DForOutWhenUnconnected=off
  wires:
  max.3/1(Out) -> Min/1
  Gain3/1 -> Mux2/4
  Gain2/1 -> Mux2/3
  Gain1/1 -> Mux2/2
  Product/1 -> max.3/Trigger
  Counter.2/1(En) -> Gain2/1, Product/1
  Mux2/1 -> Scope3/1
  Counter.1/1(En) -> Gain3/1, Product/2
  max.1/1(Out) -> max.3/1(In)
  Relational Operator/1 -> Gain1/1, Counter.2/1(Sig.In), Counter.1/1(Sig.In), max.1/Trigger
  In/1 -> Mux2/1, Relational Operator/1, max.1/1(In), Unit Delay/1
  Unit Delay/1 -> Relational Operator/2

== system FOC_PMSM/Rotor Pos. estimation/Cal. stator flux linkage/MinMax detection/Max. Det/Counter.1 ==
  Sig.In : Inport
  Constant4 : Constant  Value=10
  Constant5 : Constant
  Conter with enable : Subsystem
  Sum1 : Sum  Inputs=|-+
  En : Outport  VectorParamsAs1DForOutWhenUnconnected=off
  wires:
  Constant5/1 -> Sum1/2
  Sig.In/1 -> Sum1/1
  Conter with enable/1(Max. Reached?) -> En/1
  Sum1/1 -> Conter with enable/1(_|  |_)
  Constant4/1 -> Conter with enable/2(Max. Num)

== system FOC_PMSM/Rotor Pos. estimation/Cal. stator flux linkage/MinMax detection/Max. Det/Counter.2 ==
  Sig.In : Inport
  Constant4 : Constant  Value=5
  Conter with enable : Subsystem
  Gain : Gain  Gain=2
  Gain1 : Gain  Gain=3
  Gain2 : Gain  Gain=4
  Mux1 : Mux
  Rising edge gen. : Subsystem
  SR Latch : Subsystem
  Scope2 : Scope
  En : Outport  VectorParamsAs1DForOutWhenUnconnected=off
  wires:
  Constant4/1 -> Conter with enable/2(Max. Num)
  Sig.In/1 -> Conter with enable/1(_|  |_), Rising edge gen./1(_|  |_), Gain2/1
  Conter with enable/1(Max. Reached?) -> SR Latch/2(S), Gain1/1
  SR Latch/1(Q) -> En/1, Mux1/1
  Mux1/1 -> Scope2/1
  Rising edge gen./1(Edge) -> SR Latch/1(R), Gain/1
  Gain/1 -> Mux1/2
  Gain1/1 -> Mux1/3
  Gain2/1 -> Mux1/4

== system FOC_PMSM/Rotor Pos. estimation/Cal. stator flux linkage/MinMax detection/Max. Det/max.1 ==
  In : Inport
  Trigger : TriggerPort  TriggerType=falling  VariantControl=(inherit)
  Out : Outport  VectorParamsAs1DForOutWhenUnconnected=off
  wires:
  In/1 -> Out/1

== system FOC_PMSM/Rotor Pos. estimation/Cal. stator flux linkage/MinMax detection/Max. Det/max.3 ==
  In : Inport
  Trigger : TriggerPort  VariantControl=(inherit)
  Out : Outport  VectorParamsAs1DForOutWhenUnconnected=off
  wires:
  In/1 -> Out/1

== system FOC_PMSM/Rotor Pos. estimation/Cal. stator flux linkage/MinMax detection/Min. Det/Counter.1 ==
  Sig.In : Inport
  Constant4 : Constant  Value=10
  Constant5 : Constant
  Conter with enable : Subsystem
  Sum1 : Sum  Inputs=|-+
  En : Outport  VectorParamsAs1DForOutWhenUnconnected=off
  wires:
  Constant4/1 -> Conter with enable/2(Max. Num)
  Sum1/1 -> Conter with enable/1(_|  |_)
  Conter with enable/1(Max. Reached?) -> En/1
  Sig.In/1 -> Sum1/1
  Constant5/1 -> Sum1/2

== system FOC_PMSM/Rotor Pos. estimation/Cal. stator flux linkage/MinMax detection/Min. Det/Counter.2 ==
  Sig.In : Inport
  Constant4 : Constant  Value=5
  Conter with enable : Subsystem
  Gain : Gain  Gain=2
  Gain1 : Gain  Gain=3
  Gain2 : Gain  Gain=4
  Mux1 : Mux
  Rising edge gen. : Subsystem
  SR Latch : Subsystem
  Scope2 : Scope
  En : Outport  VectorParamsAs1DForOutWhenUnconnected=off
  wires:
  Gain2/1 -> Mux1/4
  Gain1/1 -> Mux1/3
  Gain/1 -> Mux1/2
  Rising edge gen./1(Edge) -> Gain/1, SR Latch/1(R)
  Mux1/1 -> Scope2/1
  SR Latch/1(Q) -> Mux1/1, En/1
  Conter with enable/1(Max. Reached?) -> Gain1/1, SR Latch/2(S)
  Sig.In/1 -> Gain2/1, Rising edge gen./1(_|  |_), Conter with enable/1(_|  |_)
  Constant4/1 -> Conter with enable/2(Max. Num)

== system FOC_PMSM/Rotor Pos. estimation/Cal. stator flux linkage/MinMax detection/Min. Det/max.1 ==
  In : Inport
  Trigger : TriggerPort  TriggerType=falling  VariantControl=(inherit)
  Out : Outport  VectorParamsAs1DForOutWhenUnconnected=off
  wires:
  In/1 -> Out/1

== system FOC_PMSM/Rotor Pos. estimation/Cal. stator flux linkage/MinMax detection/Min. Det/max.3 ==
  In : Inport
  Trigger : TriggerPort  VariantControl=(inherit)
  Out : Outport  VectorParamsAs1DForOutWhenUnconnected=off
  wires:
  In/1 -> Out/1

== system FOC_PMSM/Rotor Pos. estimation/Cal. stator flux linkage1/MinMax detection/Max. Det/Counter.1 ==
  Sig.In : Inport
  Constant4 : Constant  Value=10
  Constant5 : Constant
  Conter with enable : Subsystem
  Sum1 : Sum  Inputs=|-+
  En : Outport  VectorParamsAs1DForOutWhenUnconnected=off
  wires:
  Constant5/1 -> Sum1/2
  Sig.In/1 -> Sum1/1
  Conter with enable/1(Max. Reached?) -> En/1
  Sum1/1 -> Conter with enable/1(_|  |_)
  Constant4/1 -> Conter with enable/2(Max. Num)

== system FOC_PMSM/Rotor Pos. estimation/Cal. stator flux linkage1/MinMax detection/Max. Det/Counter.2 ==
  Sig.In : Inport
  Constant4 : Constant  Value=5
  Conter with enable : Subsystem
  Gain : Gain  Gain=2
  Gain1 : Gain  Gain=3
  Gain2 : Gain  Gain=4
  Mux1 : Mux
  Rising edge gen. : Subsystem
  SR Latch : Subsystem
  Scope2 : Scope
  En : Outport  VectorParamsAs1DForOutWhenUnconnected=off
  wires:
  Constant4/1 -> Conter with enable/2(Max. Num)
  Sig.In/1 -> Conter with enable/1(_|  |_), Rising edge gen./1(_|  |_), Gain2/1
  Conter with enable/1(Max. Reached?) -> SR Latch/2(S), Gain1/1
  SR Latch/1(Q) -> En/1, Mux1/1
  Mux1/1 -> Scope2/1
  Rising edge gen./1(Edge) -> SR Latch/1(R), Gain/1
  Gain/1 -> Mux1/2
  Gain1/1 -> Mux1/3
  Gain2/1 -> Mux1/4

== system FOC_PMSM/Rotor Pos. estimation/Cal. stator flux linkage1/MinMax detection/Max. Det/max.1 ==
  In : Inport
  Trigger : TriggerPort  TriggerType=falling  VariantControl=(inherit)
  Out : Outport  VectorParamsAs1DForOutWhenUnconnected=off
  wires:
  In/1 -> Out/1

== system FOC_PMSM/Rotor Pos. estimation/Cal. stator flux linkage1/MinMax detection/Max. Det/max.3 ==
  In : Inport
  Trigger : TriggerPort  VariantControl=(inherit)
  Out : Outport  VectorParamsAs1DForOutWhenUnconnected=off
  wires:
  In/1 -> Out/1

== system FOC_PMSM/Rotor Pos. estimation/Cal. stator flux linkage1/MinMax detection/Min. Det/Counter.1 ==
  Sig.In : Inport
  Constant4 : Constant  Value=10
  Constant5 : Constant
  Conter with enable : Subsystem
  Sum1 : Sum  Inputs=|-+
  En : Outport  VectorParamsAs1DForOutWhenUnconnected=off
  wires:
  Constant4/1 -> Conter with enable/2(Max. Num)
  Sum1/1 -> Conter with enable/1(_|  |_)
  Conter with enable/1(Max. Reached?) -> En/1
  Sig.In/1 -> Sum1/1
  Constant5/1 -> Sum1/2

== system FOC_PMSM/Rotor Pos. estimation/Cal. stator flux linkage1/MinMax detection/Min. Det/Counter.2 ==
  Sig.In : Inport
  Constant4 : Constant  Value=5
  Conter with enable : Subsystem
  Gain : Gain  Gain=2
  Gain1 : Gain  Gain=3
  Gain2 : Gain  Gain=4
  Mux1 : Mux
  Rising edge gen. : Subsystem
  SR Latch : Subsystem
  Scope2 : Scope
  En : Outport  VectorParamsAs1DForOutWhenUnconnected=off
  wires:
  Gain2/1 -> Mux1/4
  Gain1/1 -> Mux1/3
  Gain/1 -> Mux1/2
  Rising edge gen./1(Edge) -> Gain/1, SR Latch/1(R)
  Mux1/1 -> Scope2/1
  SR Latch/1(Q) -> Mux1/1, En/1
  Conter with enable/1(Max. Reached?) -> Gain1/1, SR Latch/2(S)
  Sig.In/1 -> Gain2/1, Rising edge gen./1(_|  |_), Conter with enable/1(_|  |_)
  Constant4/1 -> Conter with enable/2(Max. Num)

== system FOC_PMSM/Rotor Pos. estimation/Cal. stator flux linkage1/MinMax detection/Min. Det/max.1 ==
  In : Inport
  Trigger : TriggerPort  TriggerType=falling  VariantControl=(inherit)
  Out : Outport  VectorParamsAs1DForOutWhenUnconnected=off
  wires:
  In/1 -> Out/1

== system FOC_PMSM/Rotor Pos. estimation/Cal. stator flux linkage1/MinMax detection/Min. Det/max.3 ==
  In : Inport
  Trigger : TriggerPort  VariantControl=(inherit)
  Out : Outport  VectorParamsAs1DForOutWhenUnconnected=off
  wires:
  In/1 -> Out/1

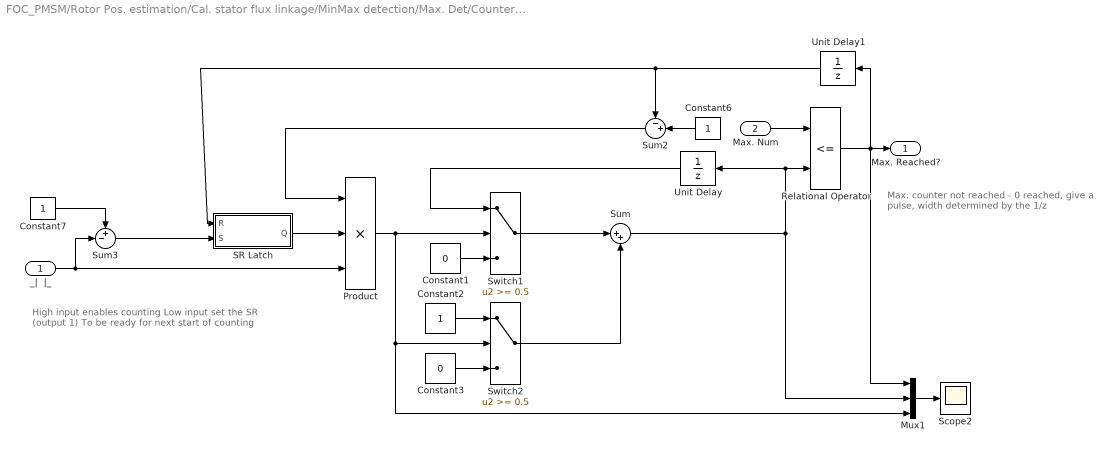
== system FOC_PMSM/Rotor Pos. estimation/Cal. stator flux linkage/MinMax detection/Max. Det/Counter.1/Conter with enable ==
  note: High input enables counting
      | Low input set the SR (output 1)
      | To be ready for next start of
      | counting
  note: Max. counter not reached - 0
      | reached, give a pulse, width
      | determined by the 1/z
  _|  |_ : Inport
  Max. Num : Inport  Port=2
  Constant1 : Constant  Value=0
  Constant2 : Constant
  Constant3 : Constant  Value=0
  Constant6 : Constant
  Constant7 : Constant
  Mux1 : Mux  Inputs=3
  Product : Product  Inputs=3  RndMeth=Zero
  Relational Operator : RelationalOperator  Operator=<=  RndMeth=Nearest
  SR Latch : Subsystem
  Scope2 : Scope
  Sum : Sum  Inputs=|++
  Sum2 : Sum  Inputs=-+|
  Sum3 : Sum  Inputs=+-|
  Switch1 : Switch  Threshold=0.5
  Switch2 : Switch  Threshold=0.5
  Unit Delay : UnitDelay  SampleTime=-1  HasFrameUpgradeWarning=on
  Unit Delay1 : UnitDelay  SampleTime=-1  HasFrameUpgradeWarning=on
  Max. Reached? : Outport  VectorParamsAs1DForOutWhenUnconnected=off
  wires:
  Constant1/1 -> Switch1/3
  Constant2/1 -> Switch2/1
  Constant3/1 -> Switch2/3
  Switch1/1 -> Sum/1
  Switch2/1 -> Sum/2
  Sum/1 -> Unit Delay/1, Relational Operator/2, Mux1/2
  Unit Delay/1 -> Switch1/1
  Max. Num/1 -> Relational Operator/1
  Relational Operator/1 -> Mux1/1, Unit Delay1/1, Max. Reached?/1
  Mux1/1 -> Scope2/1
  Sum2/1 -> Product/1
  Product/1 -> Switch1/2, Switch2/2, Mux1/3
  _|  |_/1 -> Sum3/2, Product/3
  SR Latch/1(Q) -> Product/2
  Sum3/1 -> SR Latch/2(S)
  Constant7/1 -> Sum3/1
  Constant6/1 -> Sum2/2
  Unit Delay1/1 -> Sum2/1, SR Latch/1(R)

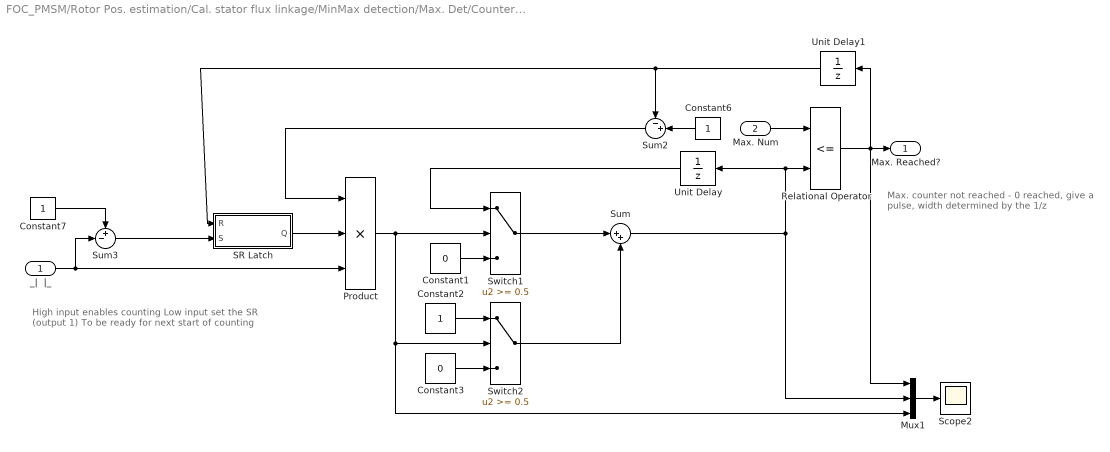
== system FOC_PMSM/Rotor Pos. estimation/Cal. stator flux linkage/MinMax detection/Max. Det/Counter.2/Conter with enable ==
  note: Max. counter not reached - 0
      | reached, give a pulse, width
      | determined by the 1/z
  note: High input enables counting
      | Low input set the SR (output 1)
      | To be ready for next start of
      | counting
  _|  |_ : Inport
  Max. Num : Inport  Port=2
  Constant1 : Constant  Value=0
  Constant2 : Constant
  Constant3 : Constant  Value=0
  Constant6 : Constant
  Constant7 : Constant
  Mux1 : Mux  Inputs=3
  Product : Product  Inputs=3  RndMeth=Zero
  Relational Operator : RelationalOperator  Operator=<=  RndMeth=Nearest
  SR Latch : Subsystem
  Scope2 : Scope
  Sum : Sum  Inputs=|++
  Sum2 : Sum  Inputs=-+|
  Sum3 : Sum  Inputs=+-|
  Switch1 : Switch  Threshold=0.5
  Switch2 : Switch  Threshold=0.5
  Unit Delay : UnitDelay  SampleTime=-1  HasFrameUpgradeWarning=on
  Unit Delay1 : UnitDelay  SampleTime=-1  HasFrameUpgradeWarning=on
  Max. Reached? : Outport  VectorParamsAs1DForOutWhenUnconnected=off
  wires:
  Unit Delay1/1 -> SR Latch/1(R), Sum2/1
  Constant6/1 -> Sum2/2
  Constant7/1 -> Sum3/1
  Sum3/1 -> SR Latch/2(S)
  SR Latch/1(Q) -> Product/2
  _|  |_/1 -> Product/3, Sum3/2
  Product/1 -> Mux1/3, Switch2/2, Switch1/2
  Sum2/1 -> Product/1
  Mux1/1 -> Scope2/1
  Relational Operator/1 -> Max. Reached?/1, Unit Delay1/1, Mux1/1
  Max. Num/1 -> Relational Operator/1
  Unit Delay/1 -> Switch1/1
  Sum/1 -> Mux1/2, Relational Operator/2, Unit Delay/1
  Switch2/1 -> Sum/2
  Switch1/1 -> Sum/1
  Constant3/1 -> Switch2/3
  Constant2/1 -> Switch2/1
  Constant1/1 -> Switch1/3

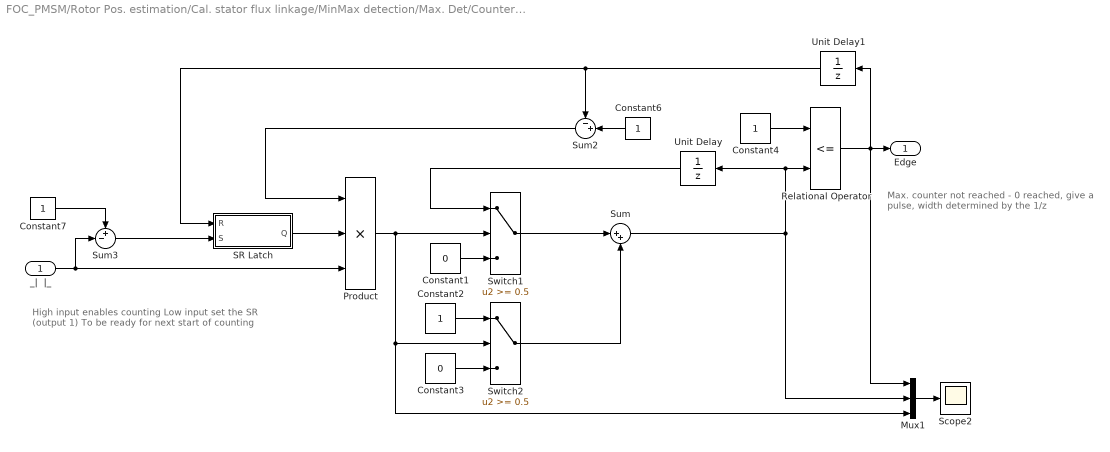
== system FOC_PMSM/Rotor Pos. estimation/Cal. stator flux linkage/MinMax detection/Max. Det/Counter.2/Rising edge gen. ==
  note: High input enables counting
      | Low input set the SR (output 1)
      | To be ready for next start of
      | counting
  note: Max. counter not reached - 0
      | reached, give a pulse, width
      | determined by the 1/z
  _|  |_ : Inport
  Constant1 : Constant  Value=0
  Constant{2,4,6..7} (4 alike) : Constant
  Constant3 : Constant  Value=0
  Mux1 : Mux  Inputs=3
  Product : Product  Inputs=3  RndMeth=Zero
  Relational Operator : RelationalOperator  Operator=<=  RndMeth=Nearest
  SR Latch : Subsystem
  Scope2 : Scope
  Sum : Sum  Inputs=|++
  Sum2 : Sum  Inputs=-+|
  Sum3 : Sum  Inputs=+-|
  Switch1 : Switch  Threshold=0.5
  Switch2 : Switch  Threshold=0.5
  Unit Delay : UnitDelay  SampleTime=-1  HasFrameUpgradeWarning=on
  Unit Delay1 : UnitDelay  SampleTime=-1  HasFrameUpgradeWarning=on
  Edge : Outport  VectorParamsAs1DForOutWhenUnconnected=off
  wires:
  Constant1/1 -> Switch1/3
  Constant2/1 -> Switch2/1
  Constant3/1 -> Switch2/3
  Switch1/1 -> Sum/1
  Switch2/1 -> Sum/2
  Sum/1 -> Unit Delay/1, Relational Operator/2, Mux1/2
  Unit Delay/1 -> Switch1/1
  Constant4/1 -> Relational Operator/1
  Relational Operator/1 -> Mux1/1, Unit Delay1/1, Edge/1
  Mux1/1 -> Scope2/1
  Sum2/1 -> Product/1
  Product/1 -> Switch1/2, Switch2/2, Mux1/3
  _|  |_/1 -> Sum3/2, Product/3
  SR Latch/1(Q) -> Product/2
  Sum3/1 -> SR Latch/2(S)
  Constant7/1 -> Sum3/1
  Constant6/1 -> Sum2/2
  Unit Delay1/1 -> Sum2/1, SR Latch/1(R)

== system FOC_PMSM/Rotor Pos. estimation/Cal. stator flux linkage/MinMax detection/Max. Det/Counter.2/SR Latch ==
  R : Inport
  S : Inport  Port=2
  Constant2 : Constant
  Constant4 : Constant  Value=0
  Constant5 : Constant  Value=0
  Multiport Switch : MultiPortSwitch  Inputs=4
  Mux1 : Mux  Inputs=2
  Selcect : Fcn  Expr=(1-u(1))*(1-u(2))+2*(1-u(1))*u(2)+3*u(1)*(1-u(2))+4*u(1)*u(2)
  Unit Delay2 : UnitDelay  SampleTime=-1  HasFrameUpgradeWarning=on
  Q : Outport  VectorParamsAs1DForOutWhenUnconnected=off
  wires:
  S/1 -> Mux1/2
  R/1 -> Mux1/1
  Constant5/1 -> Multiport Switch/5
  Constant4/1 -> Multiport Switch/4
  Constant2/1 -> Multiport Switch/3
  Unit Delay2/1 -> Multiport Switch/2
  Mux1/1 -> Selcect/1
  Selcect/1 -> Multiport Switch/1
  Multiport Switch/1 -> Unit Delay2/1, Q/1
